simulink model "System2021BB"  (R2021b)
settings: Solver=VariableStepAuto  StartTime=0.0  StopTime=20  RelTol=1e-3
values from neighbouring files (symbols this model uses):
  Cap_num = num_cells    (= 10)    [Model_Param.m]
  Cap_SC = cap/num_cells    (= 150)    [Model_Param.m]
  Sc_maxV = num_cells*MaxV    (= 38)    [Model_Param.m]
  V_bus = 60    [Model_Param.m]
undefined symbols (not defined in the file or in its folder): Ion, Lithium
libraries: spsSeriesRLCBranchLib x6, spsMosfetLib x4, spsCurrentMeasurementLib x2, slpidlib x2, eePwmGenerator x2, spsIdealSwitchLib x2, spsBatteryLib x1, spsSupercapacitorLib x1, spsDCVoltageSourceLib x1, simulink x1, spspowerguiLib x1
settings Model: Creator=mariotilocca  LastModifiedBy=mariotilocca
settings DebuggingCC: UnconnectedInputMsg=none  UnconnectedOutputMsg=none  UnconnectedLineMsg=none
settings RTWCC: DLArmComputeVersion=20.02.1

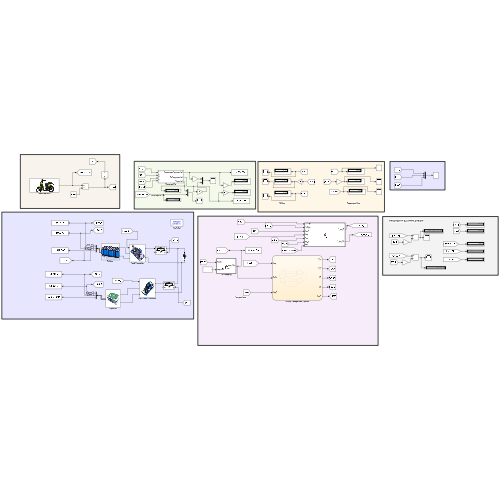
[thumbnail: Simulink's stored preview of the top-level diagram]
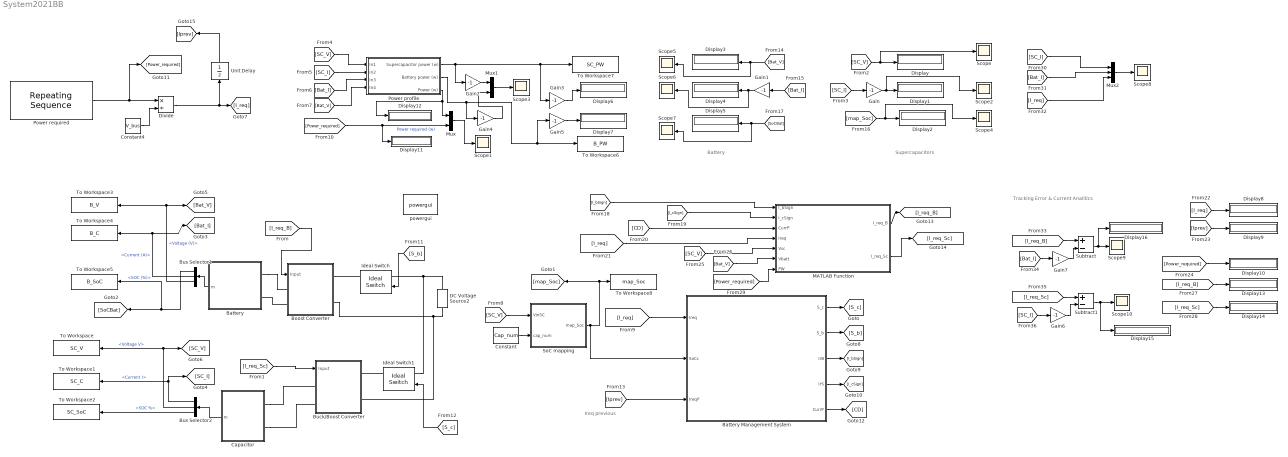
== system System2021BB ==
  note: Tracking Error & Current Analitics
  note: Ireq previous
  note: Supercapacitors
  note: Battery
  Battery : Subsystem
      mask Display: image('$imagefile'); % Use "Edit Image" on toolstrip to change.
  Battery Management System : Stateflow chart  TreatAsAtomicUnit=on
  Boost Converter : Subsystem
      mask Display: image('$imagefile'); % Use "Edit Image" on toolstrip to change.
  Buck/Boost Converter : Subsystem
      mask Display: image('$imagefile'); % Use "Edit Image" on toolstrip to change.
  Bus Selector1 : BusSelector  OutputSignals=SOC (%),Current (A),Voltage (V)
  Bus Selector2 : BusSelector  OutputSignals=Current I,Voltage V,SOC %
  Capacitor : Subsystem
      mask Display: image('$imagefile'); % Use "Edit Image" on toolstrip to change.
  Constant : Constant  Value=Cap_num
  Constant4 : Constant  Value=V_bus
  DC Voltage Source2 : spsDCVoltageSourceLib/DC Voltage Source  Amplitude=60  Measurements=Voltage
  Display{,1..16} (17 alike) : Display
  Divide : Product  Inputs=*/
  Gain{,1..7} (8 alike) : Gain  Gain=-1
  Ideal Switch : spsIdealSwitchLib/Ideal Switch  Ron=0.001  Lon=0  IC=0  Rs=1e5  Cs=inf  Measurements=on
  Ideal Switch1 : spsIdealSwitchLib/Ideal Switch  Ron=0.001  Lon=0  IC=0  Rs=1e5  Cs=inf  Measurements=on
  MATLAB Function : MATLAB Function  TreatAsAtomicUnit=on
  Mux : Mux  Inputs=2
  Mux1 : Mux  Inputs=2
  Mux2 : Mux  Inputs=3
  Power profile : Subsystem
  Power required : simulink/Sources/Repeating Sequence  rep_seq_t=simLen  rep_seq_y=PwR_profile  mask(Repeating table){}
      mask Display: image('$imagefile'); % Use "Edit Image" on toolstrip to change.
  Scope{,1..10} (11 alike) : Scope
  SoC mapping : MATLAB Function  TreatAsAtomicUnit=on
  Subtract : Sum  Inputs=+-
  Subtract1 : Sum  Inputs=+-
  To Workspace : ToWorkspace  VariableName=SC_V  SaveFormat=Timeseries  SampleTime=-1
  To Workspace1 : ToWorkspace  VariableName=SC_C  SaveFormat=Timeseries  SampleTime=-1
  To Workspace2 : ToWorkspace  VariableName=SC_SoC  SaveFormat=Timeseries  SampleTime=-1
  To Workspace3 : ToWorkspace  VariableName=B_V  SaveFormat=Timeseries  SampleTime=-1
  To Workspace4 : ToWorkspace  VariableName=B_C  SaveFormat=Timeseries  SampleTime=-1
  To Workspace5 : ToWorkspace  VariableName=B_SoC  SaveFormat=Timeseries  SampleTime=-1
  To Workspace6 : ToWorkspace  VariableName=B_PW  SaveFormat=Timeseries  SampleTime=-1
  To Workspace7 : ToWorkspace  VariableName=SC_PW  SaveFormat=Timeseries  SampleTime=-1
  To Workspace8 : ToWorkspace  VariableName=map_Soc  SaveFormat=Timeseries  SampleTime=-1
  Unit Delay : UnitDelay  SampleTime=-1  HasFrameUpgradeWarning=on
  powergui : spspowerguiLib/powergui  Priority=1  SimulationMode=Discrete  SampleTime=10e-5  frequency=60  Iterations=50  frequencyindice=0  Pbase=100e6  ErrMax=1e-4  UnitsV=kV  UnitsW=MW  buscounter=0  FunctionMessages=off  echomessages=off  EnableUseOfTLC=off  CurrentSourceSwitches=off  DisableSnubberDevices=off  DisableRonSwitches=off  DisableVfSwitches=off  DisplayEquations=off  AutomaticDiscreteSolvers=off  SolverType=Tustin/Backward Euler (TBE)  Interpol=off  ExternalGateDelay=off  methode=off  Ts=0  x0status=blocks  SPID=off  SwTol=0  HookPort=off  NonlinearTolerance=1e-4  nMaxIteration=100  ContinueOnMaxIteration=off  RestoreLinks=warning  ResistiveCurrentMeasurement=off  Frange=[0:1:1000]  Ylog=on  Xlog=on  ShowGrid=on  save=on  variable=ZDa  structure=donnee  ZoomFFT=off  StartTime=0.0  cycles=1  DisplayStyle=1  fundamental=60  FreqAxis=off  MaxFrequency=1000  frequencyindicesteady=10  RmsSteady=1  display=off
  wires:
  Bus Selector2/3 -> To Workspace2/1  "<SOC %>"
  Bus Selector2/1 -> [SC_I], To Workspace1/1  "<Current I>"
  Bus Selector1/2 -> [Bat_I], To Workspace4/1  "<Current (A)>"
  [Power_required] -> Mux/2, Display11/1  "Power required (w)"
  Bus Selector2/2 -> To Workspace/1, [SC_V]  "<Voltage V>"
  Battery/1(m) -> Bus Selector1/1
  Capacitor/1(m) -> Bus Selector2/1
  Power profile/2(Battery power (w)) -> Gain4/1, To Workspace6/1, Gain5/1
  Power profile/1(Supercapacitor power (w)) -> To Workspace7/1, Gain3/1, Gain2/1
  [SC_V] -> Power profile/1(In1)
  [SC_I] -> Power profile/2(In2)
  [Bat_I] -> Power profile/3(In3)
  [Bat_V] -> Power profile/4(In4)
  Power profile/3(Power (w)) -> Mux/1, Display12/1
  [SC_V] -> SoC mapping/1(VinSC)
  SoC mapping/1(map_Soc) -> To Workspace8/1, [map_Soc], Battery Management System/2(SoCc)
  Constant/1 -> SoC mapping/2(cap_num)
  [I_req_B] -> Boost Converter/1(Input)
  [I_req_Sc] -> Buck/Boost Converter/1(Input)
  Constant4/1 -> Divide/2
  [SC_V] -> Scope/1, Display/1
  [Bat_V] -> Scope5/1, Display3/1
  [map_Soc] -> Scope4/1, Display2/1
  [SoCBat] -> Scope7/1, Display5/1
  Power required/1 -> [Power_required], Divide/1
  Battery Management System/1(S_c) -> [S_c]
  Battery Management System/2(S_b) -> [S_b]
  [S_b] -> Ideal Switch/1
  [S_c] -> Ideal Switch1/1
  Battery Management System/3(IrB) -> [I_bSign]
  Battery Management System/4(IrS) -> [I_cSign]
  Battery Management System/5(CurrP) -> [CD]
  MATLAB Function/1(I_req_B) -> [I_req_B]
  MATLAB Function/2(I_req_Sc) -> [I_req_Sc]
  [I_bSign] -> MATLAB Function/1(I_bSign)
  [I_cSign] -> MATLAB Function/2(I_cSign)
  [CD] -> MATLAB Function/3(CurrP)
  [I_req] -> MATLAB Function/4(Ireq)
  Unit Delay/1 -> [Iprev]
  [I_req] -> Display8/1
  [Iprev] -> Display9/1
  [Power_required] -> Display10/1
  [SC_V] -> MATLAB Function/5(Vsc)
  [Bat_V] -> MATLAB Function/6(Vbatt)
  [I_req_B] -> Display13/1
  [I_req_Sc] -> Display14/1
  [Power_required] -> MATLAB Function/7(PW)
  [SC_I] -> Gain/1
  Gain/1 -> Scope2/1, Display1/1
  Gain1/1 -> Scope6/1, Display4/1
  [Bat_I] -> Gain1/1
  Bus Selector1/3 -> To Workspace3/1, [Bat_V]  "<Voltage (V)>"
  Bus Selector1/1 -> To Workspace5/1, [SoCBat]  "<SOC (%)>"
  Mux/1 -> Scope1/1
  Mux1/1 -> Scope3/1
  Mux2/1 -> Scope8/1
  [I_req] -> Mux2/3
  Divide/1 -> Unit Delay/1, [I_req]
  [I_req] -> Battery Management System/1(Ireq)
  [Iprev] -> Battery Management System/3(IreqP)
  [SC_I] -> Mux2/1
  [Bat_I] -> Mux2/2
  Gain2/1 -> Mux1/1
  Gain3/1 -> Display6/1
  Gain4/1 -> Mux1/2
  Gain5/1 -> Display7/1
  [I_req_B] -> Subtract/1
  Subtract/1 -> Display16/1, Scope9/1
  [I_req_Sc] -> Subtract1/1
  Subtract1/1 -> Display15/1, Scope10/1
  [SC_I] -> Gain6/1
  Gain6/1 -> Subtract1/2
  [Bat_I] -> Gain7/1
  Gain7/1 -> Subtract/2
  connections:
  Ideal Switch/LConn1 -- Ideal Switch1/LConn1 -- DC Voltage Source2/RConn1
  DC Voltage Source2/LConn1 -- Boost Converter/RConn2 -- Buck/Boost Converter/RConn2
  Boost Converter/LConn2 -- Battery/LConn2
  Capacitor/LConn1 -- Buck/Boost Converter/LConn1
  Capacitor/LConn2 -- Buck/Boost Converter/LConn2
  Battery/LConn1 -- Boost Converter/LConn1
  Ideal Switch/RConn1 -- Boost Converter/RConn1
  Ideal Switch1/RConn1 -- Buck/Boost Converter/RConn1

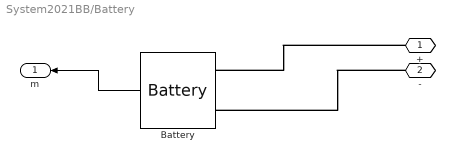
== system System2021BB/Battery ==
  Battery : spsBatteryLib/Battery  BatType=Lithium-Ion  ShowTempParam=off  ThermalPreset=no  ShowAgeParam=off  NomV=Batt_NV  NomQ=Batt_Cap  SOC=Init_Batt_SoC  Batt_Tr=1  PresetModel=on  MaxQ=76  MinV=33.3  FullV=51.681  Dis_rate=33.0435  R=0.0058421  Normal_OP=68.7304  expZone="[47.9691      3.73391]"  current=[6.5 14 20]  Units=Time  Tci=20  NomT=20  T2=-30  MaxQ2=4.8  FullV2=7.1  Normal_OP2=5.655  expZone2="[6.58           1]"  Rca=0.6  ti=2000  Dp=0  Neq0=0  Tsim=1e6  Ta1=25  Qeol=5.4*0.9  Reol=0.013333*1.2  Char_age=[2.3478, 3]  Dis_age=[2.3478, 10]  N1=1500  N2=10500  N3=1000  N4=1400  Ta2=45  N5=950
  + : PMIOPort  Side=Left
  - : PMIOPort  Port=2  Side=Left
  m : Outport
  wires:
  Battery/1 -> m/1
  connections:
  -/RConn1 -- Battery/LConn2
  +/RConn1 -- Battery/LConn1

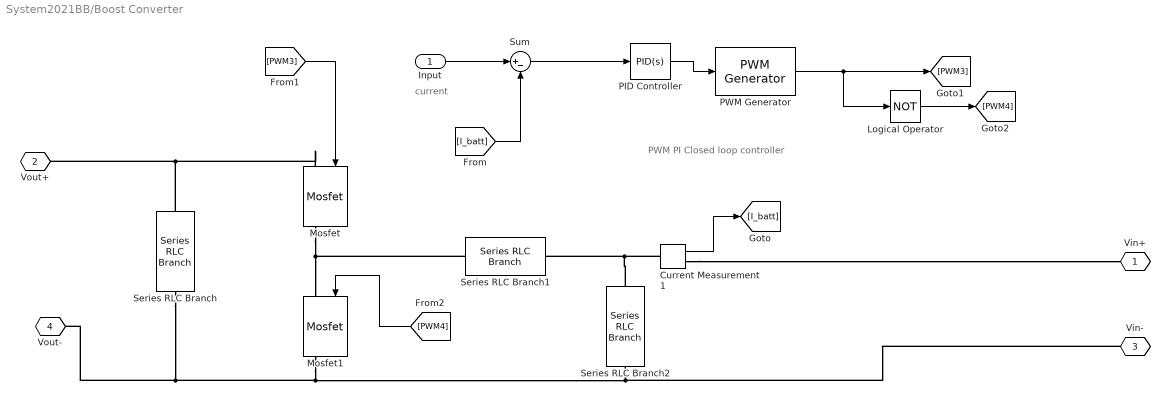
== system System2021BB/Boost Converter ==
  note: current
  note: PWM PI Closed loop controller
  Input : Inport
  Current Measurement1 : spsCurrentMeasurementLib/Current Measurement  PhasorSimulation=off  OutputType=Complex  PSBequivalent=0
  Logical Operator : Logic  Operator=NOT  AllPortsSameDT=off  OutDataTypeStr=boolean
  Mosfet : spsMosfetLib/Mosfet  Ron=0.1  Lon=0  Rd=0.01  Vfd=0  IC=0  Rs=1e5  Cs=inf  Measurements=on
  Mosfet1 : spsMosfetLib/Mosfet  Ron=0.1  Lon=0  Rd=0.01  Vfd=0  IC=0  Rs=1e5  Cs=inf  Measurements=on
  PID Controller : slpidlib/PID Controller  Controller=PID  Form=Parallel  TimeDomain=Continuous-time  UseExternalTs=off  SampleTime=-1  IntegratorMethod=Forward Euler  FilterMethod=Forward Euler  ControllerParametersSource=internal  P=2.5  I=25  D=0.2  UseFilter=on  N=100  TunerSelectOption=Transfer Function Based (PID Tuner App)  InitialConditionSource=internal  InitialConditionForIntegrator=0  InitialConditionForFilter=0  DifferentiatorICPrevScaledInput=0  ExternalReset=none  TrackingMode=off  Kt=1  LimitOutput=on  SatLimitsSource=internal  UpperSaturationLimit=0.99  LowerSaturationLimit=0  LinearizeAsGain=on  AntiWindupMode=none  Kb=1  POutMin=[]  POutMax=[]  IOutMin=[]  IOutMax=[]  DOutMin=[]  DOutMax=[]  NOutMin=[]  NOutMax=[]  SumOutMin=[]  SumOutMax=[]  SaturationOutMin=[]  SaturationOutMax=[]  PParamMin=[]  PParamMax=[]  IParamMin=[]  IParamMax=[]  DParamMin=[]  DParamMax=[]  NParamMin=[]  NParamMax=[]  KbParamMin=[]  KbParamMax=[]  KtParamMin=[]  KtParamMax=[]  KbOutMin=[]  KbOutMax=[]  KtOutMin=[]  KtOutMax=[]  IntegratorOutMin=[]  IntegratorOutMax=[]  FilterOutMin=[]  FilterOutMax=[]  SumI1OutMin=[]  SumI1OutMax=[]  SumI2OutMin=[]  SumI2OutMax=[]  SumI3OutMin=[]  SumI3OutMax=[]  SumI4OutMin=[]  SumI4OutMax=[]  SumDOutMin=[]  SumDOutMax=[]  DifferentiatorOutMin=[]  DifferentiatorOutMax=[]  FilterDiffOutCoefMin=[]  FilterDiffOutCoefMax=[]  ReciprocalOutMin=[]  ReciprocalOutMax=[]  SumDenOutMin=[]  SumDenOutMax=[]  SumNumOutMin=[]  SumNumOutMax=[]  DivideOutMin=[]  DivideOutMax=[]  UdiffTsProdOutMin=[]  UdiffTsProdOutMax=[]  NTsProdOutMin=[]  NTsProdOutMax=[]  UintegralTsProdOutMin=[]  UintegralTsProdOutMax=[]  UngainTsProdOutMin=[]  UngainTsProdOutMax=[]  IntegratorContinuousStateAttributes=''  IntegratorStateMustResolveToSignalObject=off  IntegratorRTWStateStorageClass=Auto  FilterContinuousStateAttributes=''  FilterStateMustResolveToSignalObject=off  FilterRTWStateStorageClass=Auto  ParallelPVariant=InternalParameters  IdealPVariant=Disabled  IVariant=InternalParameters  DVariant=InternalParameters  IntegratorVariant=Continuous  SatVariant=Enabled  AWVariant=Passthrough  PCopyVariant=Disabled  TRVariant=Disabled  FdbkBlocksVariant=Forward  IdealPFdbkVariant=Disabled  SatFdbkVariant=Disabled  DerivativeFilterVariant=ContFilter  NVariant=InternalParameters  NCopyVariant=Disabled  FilterICVariant=InternalICsFilter  IntegratorICVariant=InternalICs  ExternalResetVariant=Disabled  TRSumVariant=Passthrough  SumFdbkVariant=Disabled  SumVariant=Sum_PID  TsampFilterVariant=InternalTs  TsampNgainVariant=Passthrough  TsampIntegralVariant=Passthrough  ExternalSaturationOutDataTypeStr=Inherit: Same as second input
  PWM Generator : eePwmGenerator/PWM Generator  CarrCount=Up  Tper=1/5000  Tdelay=0  Ts=2.5e-6
  Series RLC Branch : spsSeriesRLCBranchLib/Series RLC Branch  LConnTagsString=__new0  RConnTagsString=__new0  BranchType=RC  Resistance=0.00001  Inductance=1e-3  SetiL0=off  InitialCurrent=0  Capacitance=1000e-6  Setx0=off  InitialVoltage=0  Measurements=None
  Series RLC Branch1 : spsSeriesRLCBranchLib/Series RLC Branch  LConnTagsString=__new0  RConnTagsString=__new0  BranchType=L  Resistance=1  Inductance=10e-3  SetiL0=off  InitialCurrent=0  Capacitance=1e-6  Setx0=off  InitialVoltage=0  Measurements=None
  Series RLC Branch2 : spsSeriesRLCBranchLib/Series RLC Branch  LConnTagsString=__new0  RConnTagsString=__new0  BranchType=RC  Resistance=0.00001  Inductance=1e-3  SetiL0=off  InitialCurrent=0  Capacitance=20e-6  Setx0=off  InitialVoltage=0  Measurements=None
  Sum : Sum  Inputs=|+-
  Vin+ : PMIOPort  Tag=PMCPort  Side=Left
  Vout+ : PMIOPort  Tag=PMCPort  Port=2  Side=Right
  Vin- : PMIOPort  Tag=PMCPort  Port=3  Side=Left
  Vout- : PMIOPort  Tag=PMCPort  Port=4  Side=Right
  wires:
  Input/1 -> Sum/1
  Current Measurement1/1 -> [I_batt]
  PID Controller/1 -> PWM Generator/1
  [PWM3] -> Mosfet/1
  [I_batt] -> Sum/2
  PWM Generator/1 -> [PWM3], Logical Operator/1
  Sum/1 -> PID Controller/1
  [PWM4] -> Mosfet1/1
  Logical Operator/1 -> [PWM4]
  connections:
  Series RLC Branch2/RConn1 -- Vout-/RConn1 -- Series RLC Branch/RConn1 -- Mosfet1/RConn1 -- Vin-/RConn1
  Series RLC Branch1/RConn1 -- Series RLC Branch2/LConn1 -- Current Measurement1/LConn1
  Series RLC Branch/LConn1 -- Mosfet/LConn1 -- Vout+/RConn1
  Mosfet/RConn1 -- Mosfet1/LConn1 -- Series RLC Branch1/LConn1
  Current Measurement1/RConn1 -- Vin+/RConn1

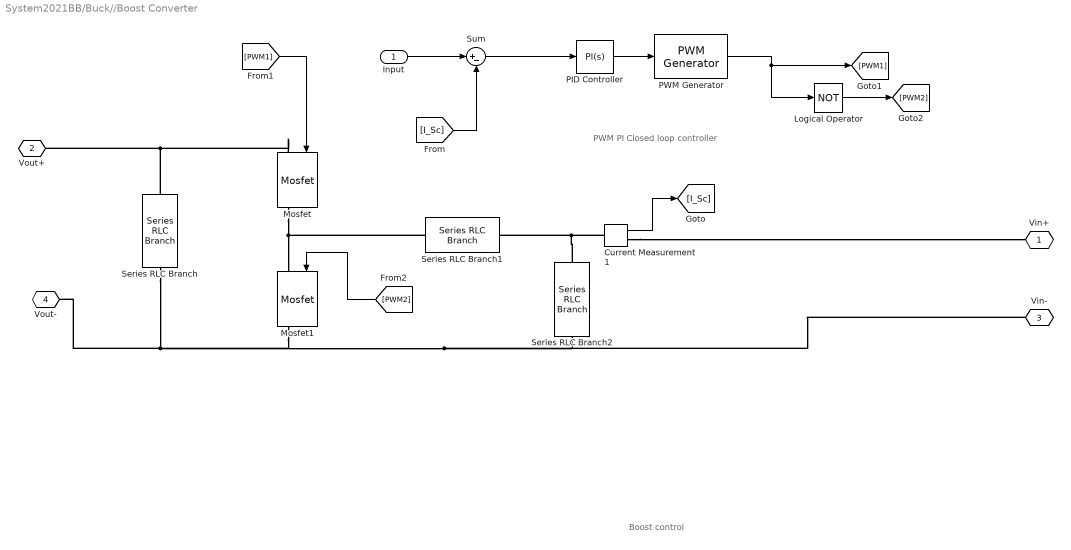
== system System2021BB/Buck//Boost Converter ==
  note: PWM PI Closed loop controller
  note: Boost control
  Input : Inport
  Current Measurement1 : spsCurrentMeasurementLib/Current Measurement  PhasorSimulation=off  OutputType=Complex  PSBequivalent=0
  Logical Operator : Logic  Operator=NOT  AllPortsSameDT=off  OutDataTypeStr=boolean
  Mosfet : spsMosfetLib/Mosfet  Ron=0.1  Lon=0  Rd=0.01  Vfd=0  IC=0  Rs=1e5  Cs=inf  Measurements=on
  Mosfet1 : spsMosfetLib/Mosfet  Ron=0.1  Lon=0  Rd=0.01  Vfd=0  IC=0  Rs=1e5  Cs=inf  Measurements=on
  PID Controller : slpidlib/PID Controller  Controller=PI  Form=Parallel  TimeDomain=Continuous-time  UseExternalTs=off  SampleTime=-1  IntegratorMethod=Forward Euler  FilterMethod=Forward Euler  ControllerParametersSource=internal  P=1.5  I=10  D=0  UseFilter=on  N=100  TunerSelectOption=Transfer Function Based (PID Tuner App)  InitialConditionSource=internal  InitialConditionForIntegrator=0  InitialConditionForFilter=0  DifferentiatorICPrevScaledInput=0  ExternalReset=none  TrackingMode=off  Kt=1  LimitOutput=on  SatLimitsSource=internal  UpperSaturationLimit=0.95  LowerSaturationLimit=0  LinearizeAsGain=on  AntiWindupMode=none  Kb=1  POutMin=[]  POutMax=[]  IOutMin=[]  IOutMax=[]  DOutMin=[]  DOutMax=[]  NOutMin=[]  NOutMax=[]  SumOutMin=[]  SumOutMax=[]  SaturationOutMin=[]  SaturationOutMax=[]  PParamMin=[]  PParamMax=[]  IParamMin=[]  IParamMax=[]  DParamMin=[]  DParamMax=[]  NParamMin=[]  NParamMax=[]  KbParamMin=[]  KbParamMax=[]  KtParamMin=[]  KtParamMax=[]  KbOutMin=[]  KbOutMax=[]  KtOutMin=[]  KtOutMax=[]  IntegratorOutMin=[]  IntegratorOutMax=[]  FilterOutMin=[]  FilterOutMax=[]  SumI1OutMin=[]  SumI1OutMax=[]  SumI2OutMin=[]  SumI2OutMax=[]  SumI3OutMin=[]  SumI3OutMax=[]  SumI4OutMin=[]  SumI4OutMax=[]  SumDOutMin=[]  SumDOutMax=[]  DifferentiatorOutMin=[]  DifferentiatorOutMax=[]  FilterDiffOutCoefMin=[]  FilterDiffOutCoefMax=[]  ReciprocalOutMin=[]  ReciprocalOutMax=[]  SumDenOutMin=[]  SumDenOutMax=[]  SumNumOutMin=[]  SumNumOutMax=[]  DivideOutMin=[]  DivideOutMax=[]  UdiffTsProdOutMin=[]  UdiffTsProdOutMax=[]  NTsProdOutMin=[]  NTsProdOutMax=[]  UintegralTsProdOutMin=[]  UintegralTsProdOutMax=[]  UngainTsProdOutMin=[]  UngainTsProdOutMax=[]  IntegratorContinuousStateAttributes=''  IntegratorStateMustResolveToSignalObject=off  IntegratorRTWStateStorageClass=Auto  FilterContinuousStateAttributes=''  FilterStateMustResolveToSignalObject=off  FilterRTWStateStorageClass=Auto  ParallelPVariant=InternalParameters  IdealPVariant=Disabled  IVariant=InternalParameters  DVariant=Disabled  IntegratorVariant=Continuous  SatVariant=Enabled  AWVariant=Passthrough  PCopyVariant=Disabled  TRVariant=Disabled  FdbkBlocksVariant=Forward  IdealPFdbkVariant=Disabled  SatFdbkVariant=Disabled  DerivativeFilterVariant=Disabled  NVariant=Disabled  NCopyVariant=Disabled_SignalSpec  FilterICVariant=Disabled  IntegratorICVariant=InternalICs  ExternalResetVariant=Disabled  TRSumVariant=Passthrough  SumFdbkVariant=Disabled  SumVariant=Sum_PI  TsampFilterVariant=InternalTs  TsampNgainVariant=Passthrough  TsampIntegralVariant=Passthrough  ExternalSaturationOutDataTypeStr=Inherit: Same as second input
  PWM Generator : eePwmGenerator/PWM Generator  CarrCount=Up  Tper=1/20000  Tdelay=0  Ts=2.5e-6
  Series RLC Branch : spsSeriesRLCBranchLib/Series RLC Branch  LConnTagsString=__new0  RConnTagsString=__new0  BranchType=RC  Resistance=0.000001  Inductance=1e-3  SetiL0=off  InitialCurrent=0  Capacitance=2000e-6  Setx0=off  InitialVoltage=0  Measurements=None
  Series RLC Branch1 : spsSeriesRLCBranchLib/Series RLC Branch  LConnTagsString=__new0  RConnTagsString=__new0  BranchType=L  Resistance=1  Inductance=10e-3  SetiL0=off  InitialCurrent=0  Capacitance=1e-6  Setx0=off  InitialVoltage=0  Measurements=None
  Series RLC Branch2 : spsSeriesRLCBranchLib/Series RLC Branch  LConnTagsString=__new0  RConnTagsString=__new0  BranchType=RC  Resistance=0.000001  Inductance=1e-3  SetiL0=off  InitialCurrent=0  Capacitance=10000e-6  Setx0=off  InitialVoltage=0  Measurements=None
  Sum : Sum  Inputs=|+-
  Vin+ : PMIOPort  Tag=PMCPort  Side=Left
  Vout+ : PMIOPort  Tag=PMCPort  Port=2  Side=Right
  Vin- : PMIOPort  Tag=PMCPort  Port=3  Side=Left
  Vout- : PMIOPort  Tag=PMCPort  Port=4  Side=Right
  wires:
  Current Measurement1/1 -> [I_Sc]
  Input/1 -> Sum/1
  [I_Sc] -> Sum/2
  Sum/1 -> PID Controller/1
  PID Controller/1 -> PWM Generator/1
  PWM Generator/1 -> [PWM1], Logical Operator/1
  Logical Operator/1 -> [PWM2]
  [PWM1] -> Mosfet/1
  [PWM2] -> Mosfet1/1
  connections:
  Series RLC Branch/LConn1 -- Mosfet/LConn1 -- Vout+/RConn1
  Series RLC Branch/RConn1 -- Vin-/RConn1 -- Series RLC Branch2/RConn1 -- Mosfet1/RConn1 -- Vout-/RConn1
  Mosfet/RConn1 -- Mosfet1/LConn1 -- Series RLC Branch1/LConn1
  Series RLC Branch2/LConn1 -- Current Measurement1/LConn1 -- Series RLC Branch1/RConn1
  Current Measurement1/RConn1 -- Vin+/RConn1

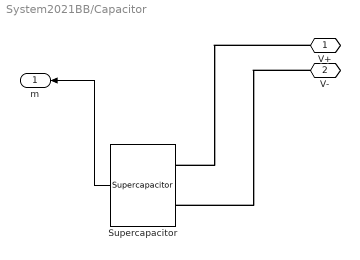
== system System2021BB/Capacitor ==
  Supercapacitor : spsSupercapacitorLib/Supercapacitor  C=Cap_SC  Rdc=Eq_RC_Sc  Voltage=Sc_maxV  Ns=Cap_num  Np=1  Vinit=Sc_init_V  Temp=Temp_Sc  PresetModel=off  EstParam=off  Nc=1  r=1e-9  epsilon=6.0208e-10  Ich=10  Vstern="[0.161  2.7  7.8]"  Self_dis=on  Ioc=20  Vself="[48  47.8  47.06  44.65]"  demandeplot=off  I=[6.5 14 20]  Units=hour  Vmax=0  If=0  deltaV=0  alpha=0  sec=0
      settings: SourceProductBaseCode=PS
  V+ : PMIOPort  Side=Left
  V- : PMIOPort  Port=2  Side=Left
  m : Outport
  wires:
  Supercapacitor/1 -> m/1
  connections:
  V+/RConn1 -- Supercapacitor/LConn1
  V-/RConn1 -- Supercapacitor/LConn2

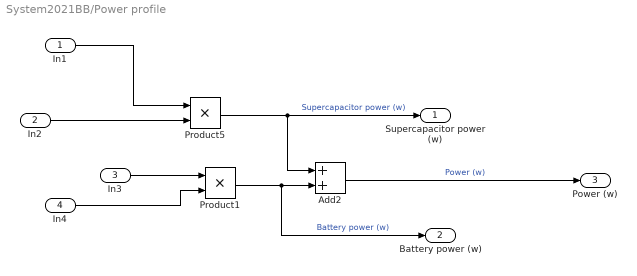
== system System2021BB/Power profile ==
  In1 : Inport
  In2 : Inport  Port=2
  In3 : Inport  Port=3
  In4 : Inport  Port=4
  Add2 : Sum
  Product1 : Product  RndMeth=Zero
  Product5 : Product  RndMeth=Zero
  Supercapacitor power (w) : Outport
  Battery power (w) : Outport  Port=2
  Power (w) : Outport  Port=3
  wires:
  In3/1 -> Product1/1
  In1/1 -> Product5/1
  Product5/1 -> Add2/1, Supercapacitor power (w)/1  "Supercapacitor power (w)"
  Add2/1 -> Power (w)/1  "Power (w)"
  Product1/1 -> Battery power (w)/1, Add2/2  "Battery power (w)"
  In4/1 -> Product1/2
  In2/1 -> Product5/2

== matlab function System2021BB/MATLAB Function ==
  data: I_bSign input; I_req_B output; I_req_Sc output; I_cSign input; CurrP input; Ireq input; Vsc input; Vbatt input; PW input
function [I_req_B, I_req_Sc] = I_flow(I_bSign, I_cSign, CurrP, Ireq, Vsc, Vbatt, PW)

I_req_B = 0;
I_req_Sc = 0;
Vbus = 60;

if  I_cSign == 1 

    I_req_Sc = -1* (Ireq *Vbus) / Vsc;
    I_req_B =0;

%     if PW <= 0 
%     I_req_Sc = 1*I_req_Sc;
%     elseif PW > 0
%         I_req_Sc = -1 *I_req_Sc;
%     end 

% elseif  I_cSign == 1 
%     I_req_Sc = (Ireq*Vbus) / Vsc;
%     I_req_B =0;
% 
%     if PW <= 0 
%     I_req_Sc = 1*I_req_Sc;
%     elseif PW > 0
%         I_req_Sc = -1 *I_req_Sc;
%     end 

elseif  I_bSign ==1 

    I_req_Sc = 0;
    I_req_B = (-1*Ireq*Vbus)/Vbatt;

%     if PW <= 0 
%     I_req_B = 1*I_req_B;
%     elseif PW > 0
%         I_req_B = -1 *I_req_B;
%     end 


elseif CurrP == 0 && I_bSign ==0 && I_cSign ==0
    I_req_Sc = 0;
    I_req_B = 0;
end 

end

== matlab function System2021BB/SoC mapping ==
  data: VinSC input; map_Soc output; cap_num input
function map_Soc = SoC_map(VinSC, cap_num)


maxR = 100;
minR = 0;

maxV = cap_num *3.8;
minV = cap_num * 2.2 ;

diffr = (VinSC - minV); 

if VinSC > maxV
    map_Soc= 100;
else 

map_Soc =((maxR-minR) /(maxV - minV)) * diffr;
end 
end

== stateflow chart System2021BB/Battery Management System ==
  note: System disconnected
  note: Discharging Supercapacitors
  state Idle
    entry:
    IrS = 0;
    IrB = 0;
    S_b = 0;
    S_c = 0;
    CurrP=0;
  state D_Sc
    entry:
    IrS =1;
    IrB = 0;
    S_b = 0;
    S_c = 1;
    CurrP =0;
  state C_Sc
    entry:
    IrS = 1;
    IrB = 0;
    S_b = 0;
    S_c = 1;
    CurrP =1;
  state D_batt
    entry:
    IrS =0;
    IrB = 1;
    S_b = 1;
    S_c = 0;
    CurrP =0;
  note: Discharging Battery pack
  note: Regenerative braking:
      | recharge supercapacitors pack
  (default) -> Idle
  Idle -> D_Sc [order 1] : [Ireq > 0 && SoCc >20]
  D_Sc -> D_batt [order 3] : [Ireq == IreqP && Ireq ~= 0 && IreqP ~=0 | SoCc < 10]
  C_Sc -> Idle [order 1] : [Ireq ==0]
  D_Sc -> Idle [order 2] : [Ireq == 0]
  D_Sc -> C_Sc [order 1] : [Ireq > 0 && IreqP < 0 && SoCc < 95 ]
  D_batt -> D_Sc [order 2] : [abs(Ireq) > abs(IreqP)]
  Idle -> C_Sc [order 2] : [Ireq < 0 && IreqP < 0]
  D_batt -> Idle [order 1] : [Ireq==0]
  C_Sc -> D_batt [order 2] : [Ireq >0 && IreqP <0]
  D_batt -> C_Sc [order 3] : [Ireq < 0 && IreqP > 0 && SoCc < 95 ]
  data: Ireq input; SoCc input; S_c output; S_b output; IrB output; IrS output; CurrP output; IreqP input
